simulink model "robustadaptivecontrola"  (R2024a)
settings: Solver=FixedStepAuto  StartTime=0.0  StopTime=8  FixedStep=0.000001  RelTol=1e-3
values from neighbouring files (symbols this model uses):
  am = 1/(Rlnom*C)    (= 53.1914893617)    [params.m]
  bm = 1    [params.m]
  C = 470e-6    (= 0.00047)    [params.m]
  k2 = 400000    [params.m]
  k3 = 700000    [params.m]
  L = 0.5e-3    (= 0.0005)    [params.m]
  R = 0.1    [params.m]
  w = 100    [params.m]
undefined symbols (not defined in the file or in its folder): alpha, E_m, epsilon, km, x2d, x3d
libraries: spsIGBTDiodeLib x6, eeTransforms x5, spsCurrentMeasurementLib x4, spsSeriesRLCBranchLib x4, spsVoltageMeasurementLib x4, spsACVoltageSourceLib x3, simulink x1, spsDCVoltageSourceLib x1, spsGroundLib x1, spsSVPWMGenerator2LevelLib x1, spsVariableResistorLib x1, spspowerguiLib x1
settings Model: Creator=CIO  LastModifiedBy=rodol
settings DebuggingCC: UnconnectedInputMsg=warning  UnconnectedOutputMsg=warning  UnconnectedLineMsg=warning
settings ModelReferenceCC: EnableRefExpFcnMdlSchedulingChecks=on
settings RTWCC: GPUComputeCapability=3.5  DLArmComputeVersion=19.05

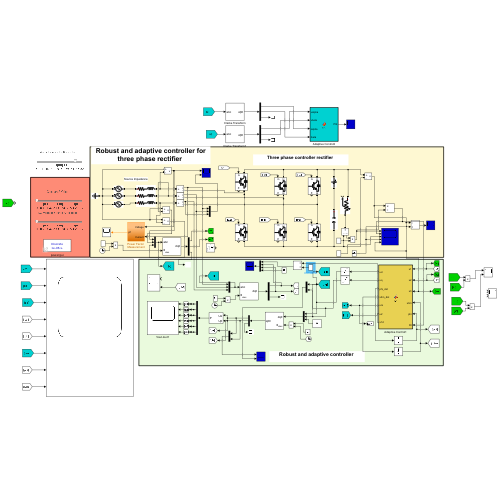
[thumbnail: Simulink's stored preview of the top-level diagram]
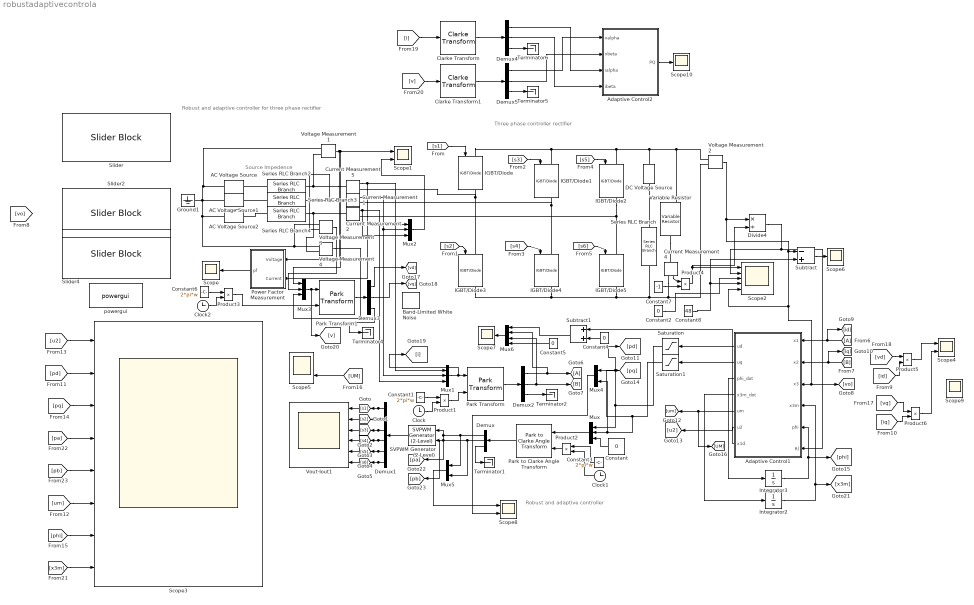
== system robustadaptivecontrola ==
  note: Source Impedence
  note: Three phase controller rectifier
  note: Robust and adaptive controller
  note: Robust and adaptive controller for three phase rectifier
  AC Voltage Source : spsACVoltageSourceLib/AC Voltage Source  Amplitude=E_m  Phase=0  Frequency=w  SampleTime=0  Measurements=None  BusType=swing  Pref=10e3  Qref=0  Qmin=-inf  Qmax=+inf
  AC Voltage Source1 : spsACVoltageSourceLib/AC Voltage Source  Amplitude=E_m  Phase=240  Frequency=w  SampleTime=0  Measurements=None  BusType=swing  Pref=10e3  Qref=0  Qmin=-inf  Qmax=+inf
  AC Voltage Source2 : spsACVoltageSourceLib/AC Voltage Source  Amplitude=E_m  Phase=120  Frequency=w  SampleTime=0  Measurements=None  BusType=swing  Pref=10e3  Qref=0  Qmin=-inf  Qmax=+inf
  Adaptive Control1 : MATLAB Function  TreatAsAtomicUnit=on
  Adaptive Control2 : MATLAB Function  TreatAsAtomicUnit=on
  Band-Limited White Noise : simulink/Sources/Band-Limited White Noise  Cov=[0.001]  Ts=0.001  seed=[23341]
  Clarke Transform : eeTransforms/Clarke Transform  PowerInvariant=off
  Clarke Transform1 : eeTransforms/Clarke Transform  PowerInvariant=off
  Clock : Clock
  Clock1 : Clock
  Clock2 : Clock
  Constant{,2,4..5} (4 alike) : Constant  Value=0
  Constant1 : Constant  Value=2*pi*w
  Constant3 : Constant  Value=2*pi*w
  Constant6 : Constant  Value=2*pi*w
  Constant7 : Constant  Value=-1
  Constant8 : Constant  Value=48
  Current Measurement{1..2,4..5} (4 alike) : spsCurrentMeasurementLib/Current Measurement  PhasorSimulation=off  OutputType=Magnitude  PSBequivalent=0
  DC Voltage Source : spsDCVoltageSourceLib/DC Voltage Source  Amplitude=0  Measurements=None
  Demux{,2..5} (5 alike) : Demux  Outputs=3
  Demux1 : Demux  Outputs=6
  Divide4 : Product  Inputs=*/
  From6 : From
  Goto6 : Goto
  Ground1 : spsGroundLib/Ground  LConnTagsString=a
  IGBT/Diode{,1..5} (6 alike) : spsIGBTDiodeLib/IGBT//Diode  Ron=1e-3  Rs=1e5  Cs=inf  Measurements=on
  Integrator2 : Integrator
  Integrator3 : Integrator
  Mux{,1..3} (4 alike) : Mux  Inputs=3
  Mux4 : Mux  Inputs=2
  Mux5 : Mux  Inputs=2
  Mux6 : Mux
  Park Transform : eeTransforms/Park Transform  AxisAlignment=D-axis  PowerInvariant=off
  Park Transform1 : eeTransforms/Park Transform  AxisAlignment=D-axis  PowerInvariant=off
  Park to Clarke Angle Transform : eeTransforms/Park to Clarke Angle Transform  AxisAlignment=D-axis
  Power Factor Measurement : Subsystem
  Product{1..6} (6 alike) : Product
  SVPWM Generator (2-Level) : spsSVPWMGenerator2LevelLib/SVPWM Generator (2-Level)  InputType=alpha-beta components  SwitchingPattern=Pattern #1  Fc=2500  ParUref=[0.8 -30 50]  Ts=0
  Saturation : Saturate  UpperLimit=50  LowerLimit=-50
  Saturation1 : Saturate  UpperLimit=25  LowerLimit=-25
  Scope{,6..7,10} (4 alike) : Scope
  Scope{1,4..5,8..9} (5 alike) : Scope  NumInputPorts=2
  Scope2 : Scope  NumInputPorts=5
  Scope3 : Scope  NumInputPorts=8
  Series RLC Branch : spsSeriesRLCBranchLib/Series RLC Branch  LConnTagsString=__new0  RConnTagsString=__new0  BranchType=C  Resistance=5  Inductance=1e-3  SetiL0=off  InitialCurrent=0  Capacitance=C  Setx0=off  InitialVoltage=0  Measurements=None
  Series RLC Branch2 : spsSeriesRLCBranchLib/Series RLC Branch  LConnTagsString=__new0  RConnTagsString=__new0  BranchType=RL  Resistance=R  Inductance=L  SetiL0=off  InitialCurrent=0  Capacitance=200e-6  Setx0=off  InitialVoltage=0  Measurements=Branch voltage and current
  Series RLC Branch3 : spsSeriesRLCBranchLib/Series RLC Branch  LConnTagsString=__new0  RConnTagsString=__new0  BranchType=RL  Resistance=R  Inductance=L  SetiL0=off  InitialCurrent=0  Capacitance=200e-6  Setx0=off  InitialVoltage=0  Measurements=Branch voltage and current
  Series RLC Branch4 : spsSeriesRLCBranchLib/Series RLC Branch  LConnTagsString=__new0  RConnTagsString=__new0  BranchType=RL  Resistance=R  Inductance=L  SetiL0=off  InitialCurrent=0  Capacitance=200e-6  Setx0=off  InitialVoltage=0  Measurements=Branch voltage and current
  Slider : SliderBlock  ScaleMin=6  ScaleMax=50
  Slider2 : SliderBlock  ScaleMax=5
  Slider4 : SliderBlock  ScaleMax=5
  Subtract : Sum  Inputs=-+
  Subtract1 : Sum
  Terminator{1..2,4..6} (5 alike) : Terminator
  Variable Resistor : spsVariableResistorLib/Variable Resistor  Rabsmin=43.5672514619883
  Voltage Measurement{1..4} (4 alike) : spsVoltageMeasurementLib/Voltage Measurement  PhasorSimulation=off  OutputType=Magnitude  PSBequivalent=0
  Vout-Iout1 : Scope  NumInputPorts=6
  powergui : spspowerguiLib/powergui  Priority=1  SimulationMode=Discrete  SampleTime=1e-6  frequency=60  Iterations=50  frequencyindice=0  Pbase=100e6  ErrMax=1e-4  UnitsV=kV  UnitsW=MW  buscounter=0  FunctionMessages=off  echomessages=off  EnableUseOfTLC=off  CurrentSourceSwitches=off  DisableSnubberDevices=off  DisableRonSwitches=off  DisableVfSwitches=off  DisplayEquations=off  AutomaticDiscreteSolvers=off  SolverType=Tustin/Backward Euler (TBE)  Interpol=off  ExternalGateDelay=off  methode=off  Ts=0  x0status=blocks  SPID=off  SwTol=0  HookPort=off  NonlinearTolerance=0  nMaxIteration=15  ContinueOnMaxIteration=off  RestoreLinks=warning  ResistiveCurrentMeasurement=off  Frange=[0:2:500]  Ylog=off  Xlog=on  ShowGrid=off  save=off  variable=ZData  structure=0  ZoomFFT=on  StartTime=0.0  cycles=1  DisplayStyle=1  fundamental=60  FreqAxis=off  MaxFrequency=1000  frequencyindicesteady=1  RmsSteady=1  display=off
  wires:
  Constant4/1 -> Subtract1/2
  Adaptive Control1/7(x1d) -> Subtract1/1
  Park to Clarke Angle Transform/1 -> Demux/1
  Clock1/1 -> Product2/2
  Product2/1 -> Park to Clarke Angle Transform/2
  Clock/1 -> Product1/2
  From6/1 -> [id], Adaptive Control1/1(x1)
  Demux2/3 -> Terminator2/1
  Divide4/1 -> Adaptive Control1/6(Rl), Scope2/2
  Product1/1 -> Park Transform/2
  Constant8/1 -> Subtract/2, Scope2/4
  Constant1/1 -> Product1/1
  Current Measurement2/1 -> Mux2/3, Mux1/3
  Constant3/1 -> Product2/1
  [s2] -> IGBT/Diode3/1
  Product4/1 -> Divide4/2, Scope2/1
  Adaptive Control1/1(ud) -> Saturation/1
  Current Measurement5/1 -> Power Factor Measurement/2(Current), Mux2/1, Mux1/1
  Mux4/1 -> Scope8/2
  [s3] -> IGBT/Diode1/1
  Adaptive Control1/6(u2) -> [u2]
  Demux1/1 -> Vout-Iout1/1, [s1]
  Mux1/1 -> [i], Park Transform/1
  Adaptive Control1/5(um) -> [UM], [um]
  Demux1/5 -> Vout-Iout1/5, [s5]
  Voltage Measurement1/1 -> Power Factor Measurement/1(Voltage), Scope1/1, Mux3/1
  Current Measurement1/1 -> Mux2/2, Mux1/2
  [B] -> [iq], Adaptive Control1/2(x2)
  Constant/1 -> Mux/3
  Saturation/1 -> Mux4/1, [pd], Mux/1
  Subtract/1 -> Scope6/1
  Current Measurement4/1 -> Product4/1
  Mux2/1 -> Scope1/2
  SVPWM Generator (2-Level)/1 -> Demux1/1
  Demux/1 -> Mux5/1, SVPWM Generator (2-Level)/1, [pa]
  [s1] -> IGBT/Diode/1
  Demux2/2 -> Mux6/3, [B]
  Constant2/1 -> Scope2/3
  [s6] -> IGBT/Diode5/1
  Demux1/2 -> Vout-Iout1/2, [s2]
  [s4] -> IGBT/Diode4/1
  Park Transform/1 -> Demux2/1
  Adaptive Control1/2(uq) -> Saturation1/1
  Voltage Measurement2/1 -> Divide4/1, [vo], Adaptive Control1/3(x3), Scope2/5, Subtract/1
  Mux/1 -> Park to Clarke Angle Transform/1
  Mux6/1 -> Scope7/1
  Demux1/4 -> Vout-Iout1/4, [s4]
  Demux/2 -> Mux5/2, [pb], SVPWM Generator (2-Level)/2
  Integrator3/1 -> [phi], Adaptive Control1/5(phi)
  Demux1/3 -> Vout-Iout1/3, [s3]
  [s5] -> IGBT/Diode2/1
  Demux1/6 -> Vout-Iout1/6, [s6]
  Adaptive Control1/3(phi_dot) -> Integrator3/1
  Saturation1/1 -> [pq], Mux4/2, Mux/2
  Demux/3 -> Terminator1/1
  Mux5/1 -> Scope8/1
  Integrator2/1 -> [x3m], Adaptive Control1/4(x3m)
  Subtract1/1 -> Mux6/1
  Adaptive Control1/4(x3m_dot) -> Integrator2/1
  Constant7/1 -> Product4/2
  Power Factor Measurement/1(pf) -> Scope/1
  [UM] -> Scope5/2
  Constant5/1 -> Mux6/4
  Demux2/1 -> Mux6/2, Goto6/1
  Mux3/1 -> [v], Park Transform1/1
  Park Transform1/1 -> Demux3/1
  Voltage Measurement3/1 -> Mux3/2
  Voltage Measurement4/1 -> Mux3/3
  Clock2/1 -> Product3/2
  Constant6/1 -> Product3/1
  Product3/1 -> Park Transform1/2
  Demux3/3 -> Terminator4/1
  Demux3/1 -> [vd]
  Demux3/2 -> [vq]
  [id] -> Product5/2
  [iq] -> Product6/2
  Product5/1 -> Scope4/1
  Product6/1 -> Scope4/2
  [vd] -> Product5/1
  [vq] -> Product6/1
  Clarke Transform/1 -> Demux4/1
  Clarke Transform1/1 -> Demux5/1
  Demux5/3 -> Terminator5/1
  Demux4/3 -> Terminator6/1
  [i] -> Clarke Transform/1
  [v] -> Clarke Transform1/1
  Demux4/1 -> Adaptive Control2/3(ialpha)
  Demux4/2 -> Adaptive Control2/4(ibeta)
  Demux5/1 -> Adaptive Control2/1(valpha)
  Demux5/2 -> Adaptive Control2/2(vbeta)
  Adaptive Control2/1(PQ) -> Scope10/1
  [u2] -> Scope3/1
  [pd] -> Scope3/2
  [pq] -> Scope3/3
  [pa] -> Scope3/4
  [pb] -> Scope3/5
  [um] -> Scope3/6
  [phi] -> Scope3/7
  [x3m] -> Scope3/8
  connections:
  IGBT/Diode/RConn1 -- IGBT/Diode3/LConn1 -- Current Measurement5/RConn1
  Current Measurement5/LConn1 -- Series RLC Branch2/RConn1 -- Voltage Measurement1/LConn2
  Current Measurement4/RConn1 -- IGBT/Diode4/RConn1 -- IGBT/Diode3/RConn1 -- IGBT/Diode5/RConn1 -- Series RLC Branch/RConn1 -- Voltage Measurement2/LConn2
  Current Measurement2/RConn1 -- IGBT/Diode2/RConn1 -- IGBT/Diode5/LConn1
  Current Measurement1/RConn1 -- IGBT/Diode1/RConn1 -- IGBT/Diode4/LConn1
  AC Voltage Source1/RConn1 -- Voltage Measurement3/LConn1 -- Voltage Measurement4/LConn1 -- AC Voltage Source2/RConn1 -- Ground1/LConn1 -- Voltage Measurement1/LConn1 -- AC Voltage Source/RConn1
  Voltage Measurement2/LConn1 -- Variable Resistor/LConn1 -- DC Voltage Source/RConn1 -- IGBT/Diode2/LConn1 -- IGBT/Diode/LConn1 -- IGBT/Diode1/LConn1
  Series RLC Branch3/LConn1 -- AC Voltage Source1/LConn1
  Variable Resistor/RConn1 -- Current Measurement4/LConn1
  Series RLC Branch4/RConn1 -- Voltage Measurement4/LConn2 -- Current Measurement2/LConn1
  Series RLC Branch3/RConn1 -- Voltage Measurement3/LConn2 -- Current Measurement1/LConn1
  Series RLC Branch2/LConn1 -- AC Voltage Source/LConn1
  Series RLC Branch4/LConn1 -- AC Voltage Source2/LConn1
  Series RLC Branch/LConn1 -- DC Voltage Source/LConn1

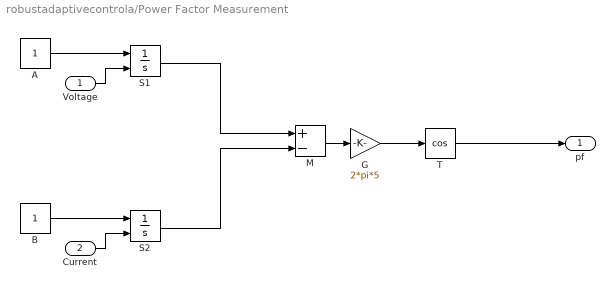
== system robustadaptivecontrola/Power Factor Measurement ==
  Voltage : Inport
  Current : Inport  Port=2
  A : Constant
  B : Constant
  G : Gain  Gain=2*pi*5
  M : Sum  Inputs=+-
  S1 : Integrator  ExternalReset=falling
  S2 : Integrator  ExternalReset=falling
  T : Trigonometry  Operator=cos
  pf : Outport
  wires:
  A/1 -> S1/1
  B/1 -> S2/1
  S1/1 -> M/1
  S2/1 -> M/2
  Voltage/1 -> S1/2
  Current/1 -> S2/2
  M/1 -> G/1
  G/1 -> T/1
  T/1 -> pf/1

== matlab function robustadaptivecontrola/Adaptive Control2 ==
  data: valpha input; PQ output; vbeta input; ialpha input; ibeta input
function PQ  = fcn(valpha,vbeta,ialpha,ibeta)


PQ = [valpha,vbeta;vbeta,-valpha]*[ialpha;ibeta];

== matlab function robustadaptivecontrola/Adaptive Control1 ==
  data: x1 input; ud output; x2 input; x3 input; x3m input; uq output; E_m parameter; C parameter; L parameter; w parameter; R parameter; x3d parameter; x2d parameter; k3 parameter; k2 parameter; epsilon parameter; phi input; phi_dot output; alpha parameter; bm parameter; km parameter; x3m_dot output; am parameter; um output; u2 output; Rl input; x1d output
function [ud , uq,phi_dot,x3m_dot,um,u2,x1d] = fcn(x1, x2, x3,x3m, E_m, C, L, w, R, x3d, x2d, k3, k2, epsilon,phi,alpha,bm,km, am, Rl)

x1d_1 = (E_m/(2*R)) + (sqrt((E_m)^2 - (8*R*x3d^2)/(3*Rl)))/(2*R);
x1d_2 = (E_m/(2*R)) - (sqrt((E_m)^2 - (8*R*x3d^2)/(3*Rl)))/(2*R);
x1d = x1d_2;

%errors
e1 = x1 - x1d;      e2 = x2 - x2d;      e3 = x3 - x3d;  

e3v =  x3 - x3m;    Qx = bm;    % theta_x = -am + 1/Rl*C ;  theta = phi +theta_x;      
theta = phi;

%controls
%para evitar singularidades agregamos el termino epsilon donde corresponda
um = (1/bm)*(x3d + (am*x3m) - km*(x3m - x3d));
x3m_dot = -am*x3m + bm*um;
phi_dot = (-alpha)*(e3v)*(x3);

uq = (2*L/((e3v + x3m)+ epsilon)) * ( (-(R/L)*(e2 + x2d)) + (w*(e1 + x1d)) + (k2*sqrt(abs(e2))*sign(e2)) );

FF = (3/(4*C))*(e2+x2d)*uq ;  

u2 = (theta*x3) + (Qx*um) - k3*sqrt(abs(e3v))*sign(e3v) - FF;

ud =  ((4*C)/3) * (u2/((e1 + x1d) + epsilon)) ;
